simulink model "SoftFishHydrodynamicControl"  (R2020a)
settings: Solver=VariableStepAuto  StartTime=0.0  StopTime=40  FixedStep=1e-4  RelTol=1e-5
InitFcn:
  | initSoftFishHydrodynamicControl
values from neighbouring files (symbols this model uses):
  A33 = 0.25 * rho * pi * robotFinHeight * gamma    (= 8.1367249728)    [initSoftFishCocontraction.m]    (also in initSoftFishCocontractionControl.m; initSoftFishHydrodynamic.m; initSoftFishHydrodynamicControl.m)
  freq = 1    [initSoftFishCocontraction.m]    (also in initSoftFishCocontractionControl.m; initSoftFishHydrodynamic.m; initSoftFishHydrodynamicControl.m)
  modelElements = 5    [initSoftFishCocontraction.m]    (also in initSoftFishCocontractionControl.m; initSoftFishHydrodynamic.m; initSoftFishHydrodynamicControl.m)
  modelPressureCoefficient = pFinal(3)    [SoftFishSingleRun.m]    (also in SoftFishSingleRunWater.m)
  modelPressureLag = pFinal(5)    [SoftFishSingleRun.m]    (also in SoftFishSingleRunWater.m)
  modelPressureStiffness = pFinal(4)    [SoftFishSingleRun.m]    (also in SoftFishSingleRunWater.m)
  NoiseLevel = 0.05    [initSoftFishCocontractionControl.m]    (also in initSoftFishHydrodynamicControl.m)
  robotBlockLength = robotLength/modelElements    (= 0.028)    [initSoftFishCocontraction.m]    (also in initSoftFishCocontractionControl.m; initSoftFishHydrodynamic.m; initSoftFishHydrodynamicControl.m)
  robotBlockRevoluteRadius = 0.5 * robotBlockLength    (= 0.014)    [initSoftFishCocontraction.m]    (also in initSoftFishCocontractionControl.m; initSoftFishHydrodynamic.m; initSoftFishHydrodynamicControl.m)
  robotChamberHeight = 2e-2    (= 0.02)    [initSoftFishCocontraction.m]    (also in initSoftFishCocontractionControl.m; initSoftFishHydrodynamic.m; initSoftFishHydrodynamicControl.m)
  robotChamberWidth = 3e-2    (= 0.03)    [initSoftFishCocontraction.m]    (also in initSoftFishCocontractionControl.m; initSoftFishHydrodynamic.m; initSoftFishHydrodynamicControl.m)
  robotFinHeight = 7e-2    (= 0.07)    [initSoftFishCocontraction.m]    (also in initSoftFishCocontractionControl.m; initSoftFishHydrodynamic.m; initSoftFishHydrodynamicControl.m)
  robotFinWidth = 0.52*1e-3    (= 0.00052)    [initSoftFishCocontraction.m]    (also in initSoftFishCocontractionControl.m; initSoftFishHydrodynamic.m; initSoftFishHydrodynamicControl.m)
  robotLength = 112e-3*1.25    (= 0.14)    [initSoftFishCocontraction.m]    (also in initSoftFishCocontractionControl.m; initSoftFishHydrodynamic.m; initSoftFishHydrodynamicControl.m)
  robotMass = 2*42e-3    (= 0.084)    [initSoftFishCocontraction.m]    (also in initSoftFishCocontractionControl.m; initSoftFishHydrodynamic.m; initSoftFishHydrodynamicControl.m)
  Setpoint1 = 0.7    [initSoftFishCocontractionControl.m]    (also in initSoftFishHydrodynamicControl.m = 0.4)
  Setpoint2 = 1.4    [initSoftFishCocontractionControl.m]    (also in initSoftFishHydrodynamicControl.m = 0.6)
  Setpoint3 = 0.5    [initSoftFishCocontractionControl.m]    (also in initSoftFishHydrodynamicControl.m = 0.4)
  SwitchTime1 = 15    [initSoftFishCocontractionControl.m]    (also in initSoftFishHydrodynamicControl.m)
  SwitchTime2 = 25    [initSoftFishCocontractionControl.m]    (also in initSoftFishHydrodynamicControl.m = 30)
undefined symbols (not defined in the file or in its folder): X, Y, Z
libraries: nesl_utility x33, sm_lib x28, fl_lib x3, simulink x2
(part 2 of 2)

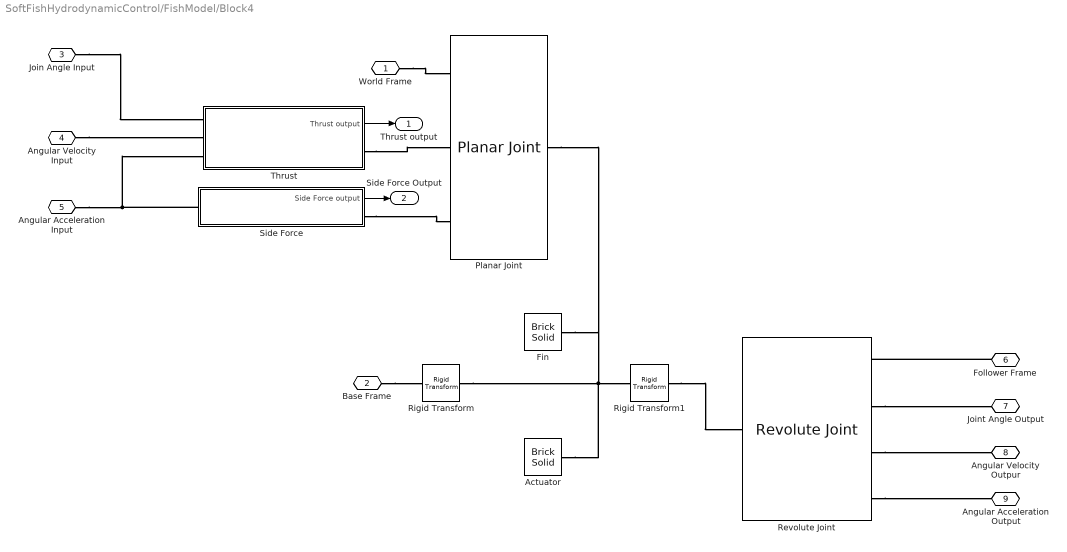
== system SoftFishHydrodynamicControl/FishModel/Block4 ==
  Actuator : sm_lib/Body Elements/Brick Solid  GraphicAmbientColor=[0.15 0.15 0.15 1.0]  BasedOnType=Mass  BrickDimensions=[robotLength/modelElements robotChamberWidth robotChamberHeight]  BrickDimensionUnits=m  CenterOfMass=[0 0 0]  CenterOfMassUnits=m  GraphicDiffuseColor=robotChamberColor  Density=1000  DensityUnits=kg/m^3  DoExposeReferenceFrame=on  GraphicEmissiveColor=[0.0 0.0 0.0 1.0]  ExportEntireGeometry=off  SerializedFrames=<Frames/>  MarkerShape=Sphere  MarkerSize=10  GraphicType=FromGeometry  InertiaType=CalculateFromGeometry  Mass=robotMass/modelElements  MassUnits=kg  MomentsOfInertia=[1 1 1]  MomentsOfInertiaUnits=kg*m^2  GraphicOpacity=1.0  ProductsOfInertia=[0 0 0]  ProductsOfInertiaUnits=kg*m^2  GraphicShininess=75  GraphicSpecularColor=[0.5 0.5 0.5 1.0]  GraphicVisPropType=SimpleVisualProperties
  Fin : sm_lib/Body Elements/Brick Solid  GraphicAmbientColor=[0.15 0.15 0.15 1.0]  BasedOnType=Density  BrickDimensions=[robotLength/modelElements robotFinWidth robotFinHeight]  BrickDimensionUnits=m  CenterOfMass=[0 0 0]  CenterOfMassUnits=m  GraphicDiffuseColor=[0.5 0.5 0.5]  Density=0  DensityUnits=kg/m^3  DoExposeReferenceFrame=on  GraphicEmissiveColor=[0.0 0.0 0.0 1.0]  ExportEntireGeometry=off  SerializedFrames=<Frames/>  MarkerShape=Sphere  MarkerSize=10  GraphicType=FromGeometry  InertiaType=CalculateFromGeometry  Mass=1  MassUnits=kg  MomentsOfInertia=[1 1 1]  MomentsOfInertiaUnits=kg*m^2  GraphicOpacity=1.0  ProductsOfInertia=[0 0 0]  ProductsOfInertiaUnits=kg*m^2  GraphicShininess=75  GraphicSpecularColor=[0.5 0.5 0.5 1.0]  GraphicVisPropType=SimpleVisualProperties
  Planar Joint : sm_lib/Joints/Planar Joint  JointMode=Normal  SenseConstraintForce=off  SenseConstraintForceX=off  SenseConstraintForceY=off  SenseConstraintForceZ=off  SenseConstraintTorque=off  SenseConstraintTorqueX=off  SenseConstraintTorqueY=off  SenseConstraintTorqueZ=off  SenseTotalForce=off  SenseTotalForceX=off  SenseTotalForceY=off  SenseTotalForceZ=off  SenseTotalTorque=off  SenseTotalTorqueX=off  SenseTotalTorqueY=off  SenseTotalTorqueZ=off  CompositeWrenchDir=FollowerOnBase  CompositeWrenchFrame=BaseFrame  PxEquilibriumPosition=0  PxEquilibriumPositionUnits=m  PxSpringStiffness=0  PxSpringStiffnessUnits=N/m  PxDampingCoefficient=0  PxDampingCoefficientUnits=N/(m/s)  PxTorqueActuationMode=InputTorque  PxMotionActuationMode=ComputedMotion  PxSensePosition=off  PxSenseVelocity=off  PxSenseAcceleration=off  PxSenseTorqueForce=off  PxSenseLowerLimitTorqueForce=off  PxSenseUpperLimitTorqueForce=off  PxLowerLimitSpecify=off  PxLowerLimitBound=-1  PxLowerLimitBoundUnits=m  PxLowerLimitStiffness=1e6  PxLowerLimitStiffnessUnits=N/m  PxLowerLimitDamping=1e3  PxLowerLimitDampingUnits=N/(m/s)  PxLowerLimitTransitionRegionWidth=1e-4  PxLowerLimitTransitionRegionWidthUnits=m  PxUpperLimitSpecify=off  PxUpperLimitBound=1  PxUpperLimitBoundUnits=m  PxUpperLimitStiffness=1e6  PxUpperLimitStiffnessUnits=N/m  PxUpperLimitDamping=1e3  PxUpperLimitDampingUnits=N/(m/s)  PxUpperLimitTransitionRegionWidth=1e-4  PxUpperLimitTransitionRegionWidthUnits=m  PxPositionTargetSpecify=off  PxPositionTargetPriority=High  PxPositionTargetValue=0  PxPositionTargetValueUnits=m  PxVelocityTargetSpecify=off  PxVelocityTargetPriority=High  PxVelocityTargetValue=0  PxVelocityTargetValueUnits=m/s  PyEquilibriumPosition=0  PyEquilibriumPositionUnits=m  PySpringStiffness=0  PySpringStiffnessUnits=N/m  PyDampingCoefficient=0  PyDampingCoefficientUnits=N/(m/s)  PyTorqueActuationMode=InputTorque  PyMotionActuationMode=ComputedMotion  PySensePosition=off  PySenseVelocity=off  PySenseAcceleration=off  PySenseTorqueForce=off  PySenseLowerLimitTorqueForce=off  PySenseUpperLimitTorqueForce=off  PyLowerLimitSpecify=off  PyLowerLimitBound=-1  PyLowerLimitBoundUnits=m  PyLowerLimitStiffness=1e6  PyLowerLimitStiffnessUnits=N/m  PyLowerLimitDamping=1e3  PyLowerLimitDampingUnits=N/(m/s)  PyLowerLimitTransitionRegionWidth=1e-4  PyLowerLimitTransitionRegionWidthUnits=m  PyUpperLimitSpecify=off  PyUpperLimitBound=1  PyUpperLimitBoundUnits=m  PyUpperLimitStiffness=1e6  PyUpperLimitStiffnessUnits=N/m  PyUpperLimitDamping=1e3  PyUpperLimitDampingUnits=N/(m/s)  PyUpperLimitTransitionRegionWidth=1e-4  PyUpperLimitTransitionRegionWidthUnits=m  PyPositionTargetSpecify=off  PyPositionTargetPriority=High  PyPositionTargetValue=0  PyPositionTargetValueUnits=m  PyVelocityTargetSpecify=off  PyVelocityTargetPriority=High  PyVelocityTargetValue=0  PyVelocityTargetValueUnits=m/s  RzEquilibriumPosition=0  RzEquilibriumPositionUnits=deg  RzSpringStiffness=0  RzSpringStiffnessUnits=N*m/deg  RzDampingCoefficient=0  RzDampingCoefficientUnits=N*m/(deg/s)  RzTorqueActuationMode=NoTorque  RzMotionActuationMode=ComputedMotion  RzSensePosition=off  RzSenseVelocity=off  RzSenseAcceleration=off  RzSenseTorqueForce=off  RzSenseLowerLimitTorqueForce=off  RzSenseUpperLimitTorqueForce=off  RzLowerLimitSpecify=off  RzLowerLimitBound=-90  RzLowerLimitBoundUnits=deg  RzLowerLimitStiffness=1e4  RzLowerLimitStiffnessUnits=N*m/deg  RzLowerLimitDamping=10  RzLowerLimitDampingUnits=N*m/(deg/s)  RzLowerLimitTransitionRegionWidth=0.1  RzLowerLimitTransitionRegionWidthUnits=deg  RzUpperLimitSpecify=off  RzUpperLimitBound=90  RzUpperLimitBoundUnits=deg  RzUpperLimitStiffness=1e4  RzUpperLimitStiffnessUnits=N*m/deg  RzUpperLimitDamping=10  RzUpperLimitDampingUnits=N*m/(deg/s)  RzUpperLimitTransitionRegionWidth=0.1  RzUpperLimitTransitionRegionWidthUnits=deg  RzPositionTargetSpecify=off  RzPositionTargetPriority=High  RzPositionTargetValue=0  RzPositionTargetValueUnits=deg  RzVelocityTargetSpecify=off  RzVelocityTargetPriority=High  RzVelocityTargetValue=0  RzVelocityTargetValueUnits=deg/s
  Revolute Joint : sm_lib/Joints/Revolute Joint  JointMode=Normal  SenseConstraintForce=off  SenseConstraintForceX=off  SenseConstraintForceY=off  SenseConstraintForceZ=off  SenseConstraintTorque=off  SenseConstraintTorqueX=off  SenseConstraintTorqueY=off  SenseConstraintTorqueZ=off  SenseTotalForce=off  SenseTotalForceX=off  SenseTotalForceY=off  SenseTotalForceZ=off  SenseTotalTorque=off  SenseTotalTorqueX=off  SenseTotalTorqueY=off  SenseTotalTorqueZ=off  CompositeWrenchDir=FollowerOnBase  CompositeWrenchFrame=BaseFrame  EquilibriumPosition=0  EquilibriumPositionUnits=deg  SpringStiffness=robotFinStiffness  SpringStiffnessUnits=N*m/rad  DampingCoefficient=0  DampingCoefficientUnits=N*m/(deg/s)  TorqueActuationMode=NoTorque  MotionActuationMode=ComputedMotion  SensePosition=on  SenseVelocity=on  SenseAcceleration=on  SenseTorqueForce=off  SenseLowerLimitTorqueForce=off  SenseUpperLimitTorqueForce=off  LowerLimitSpecify=off  LowerLimitBound=-90  LowerLimitBoundUnits=deg  LowerLimitStiffness=1e4  LowerLimitStiffnessUnits=N*m/deg  LowerLimitDamping=10  LowerLimitDampingUnits=N*m/(deg/s)  LowerLimitTransitionRegionWidth=0.1  LowerLimitTransitionRegionWidthUnits=deg  UpperLimitSpecify=off  UpperLimitBound=90  UpperLimitBoundUnits=deg  UpperLimitStiffness=1e4  UpperLimitStiffnessUnits=N*m/deg  UpperLimitDamping=10  UpperLimitDampingUnits=N*m/(deg/s)  UpperLimitTransitionRegionWidth=0.1  UpperLimitTransitionRegionWidthUnits=deg  PositionTargetSpecify=off  PositionTargetPriority=High  PositionTargetValue=0  PositionTargetValueUnits=deg  VelocityTargetSpecify=off  VelocityTargetPriority=High  VelocityTargetValue=0  VelocityTargetValueUnits=deg/s
  Rigid Transform : sm_lib/Frames and Transforms/Rigid Transform  TranslationMethod=StandardAxis  TranslationStandardOffset=robotLength*0.5/modelElements  TranslationLengthUnit=m  TranslationStandardAxis=+X  TranslationCartesianOffset=[0 0 0]  TranslationROffset=0  TranslationROffsetUnits=m  TranslationZOffset=0  TranslationZOffsetUnits=m  TranslationThetaOffset=0  TranslationThetaOffsetUnits=deg  RotationMethod=None  RotationAngleUnits=deg  RotationStandardAxis=+Z  RotationAngle=0.0  RotationArbitraryAxis=[0 0 1]  FollAlignAxisA=+X  BaseAlignAxisA=+Y  FollAlignAxisB=+Y  BaseAlignAxisB=+Z  RotationSequenceAxes=FollowerAxes  RotationSequence=XYX  RotationSequenceAngles=[0 0 0]  RotationSequenceAnglesUnits=deg  RotationMatrix=[1 0 0; 0 1 0; 0 0 1]
  Rigid Transform1 : sm_lib/Frames and Transforms/Rigid Transform  TranslationMethod=StandardAxis  TranslationStandardOffset=robotLength*0.5/modelElements  TranslationLengthUnit=m  TranslationStandardAxis=+X  TranslationCartesianOffset=[0 0 0]  TranslationROffset=0  TranslationROffsetUnits=m  TranslationZOffset=0  TranslationZOffsetUnits=m  TranslationThetaOffset=0  TranslationThetaOffsetUnits=deg  RotationMethod=None  RotationAngleUnits=deg  RotationStandardAxis=+Z  RotationAngle=0.0  RotationArbitraryAxis=[0 0 1]  FollAlignAxisA=+X  BaseAlignAxisA=+Y  FollAlignAxisB=+Y  BaseAlignAxisB=+Z  RotationSequenceAxes=FollowerAxes  RotationSequence=XYX  RotationSequenceAngles=[0 0 0]  RotationSequenceAnglesUnits=deg  RotationMatrix=[1 0 0; 0 1 0; 0 0 1]
  Side Force : Subsystem
  Thrust : Subsystem
  World Frame : PMIOPort  Side=Left
  Base Frame : PMIOPort  Port=2  Side=Left
  Join Angle Input : PMIOPort  Port=3  Side=Left
  Angular Velocity Input : PMIOPort  Port=4  Side=Left
  Angular Acceleration Input : PMIOPort  Port=5  Side=Left
  Follower Frame : PMIOPort  Port=6  Side=Right
  "Joint Angle Output " : PMIOPort  Port=7  Side=Right
  Angular Velocity Outpur : PMIOPort  Port=8  Side=Right
  Angular Acceleration Output : PMIOPort  Port=9  Side=Right
  Thrust output : Outport
  Side Force Output : Outport  Port=2
  wires:
  Thrust/1(Thrust output) -> Thrust output/1
  Side Force/1(Side Force output) -> Side Force Output/1
  connections:
  Base Frame/RConn1 -- Rigid Transform/LConn1
  Rigid Transform/RConn1 -- Actuator/RConn1 -- Rigid Transform1/LConn1 -- Planar Joint/RConn1 -- Fin/RConn1
  Rigid Transform1/RConn1 -- Revolute Joint/LConn1
  Follower Frame/RConn1 -- Revolute Joint/RConn1
  Revolute Joint/RConn2 -- "Joint Angle Output "/RConn1
  Revolute Joint/RConn3 -- Angular Velocity Outpur/RConn1
  Revolute Joint/RConn4 -- Angular Acceleration Output/RConn1
  World Frame/RConn1 -- Planar Joint/LConn1
  Angular Acceleration Input/RConn1 -- Thrust/LConn3 -- Side Force/LConn1
  Side Force/RConn1 -- Planar Joint/LConn3
  Thrust/RConn1 -- Planar Joint/LConn2
  Join Angle Input/RConn1 -- Thrust/LConn1
  Angular Velocity Input/RConn1 -- Thrust/LConn2

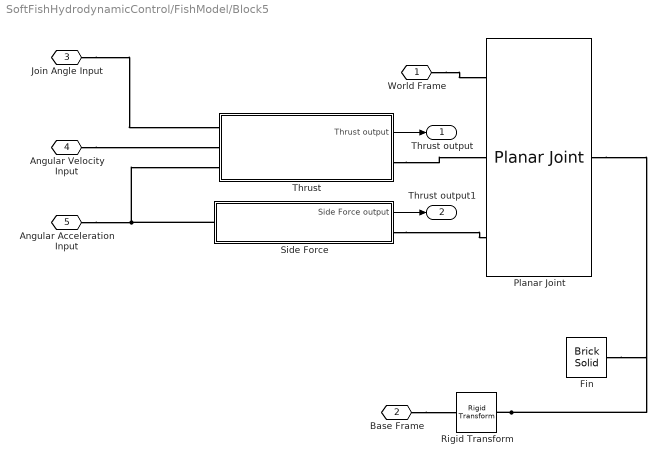
== system SoftFishHydrodynamicControl/FishModel/Block5 ==
  Fin : sm_lib/Body Elements/Brick Solid  GraphicAmbientColor=[0.15 0.15 0.15 1.0]  BasedOnType=Density  BrickDimensions=[2*robotBlockLength robotFinWidth robotFinHeight]  BrickDimensionUnits=m  CenterOfMass=[0 0 0]  CenterOfMassUnits=m  GraphicDiffuseColor=[0.5 0.5 0.5]  Density=0.92  DensityUnits=g/cm^3  DoExposeReferenceFrame=on  GraphicEmissiveColor=[0.0 0.0 0.0 1.0]  ExportEntireGeometry=off  SerializedFrames=<Frames/>  MarkerShape=Sphere  MarkerSize=10  GraphicType=FromGeometry  InertiaType=CalculateFromGeometry  Mass=1  MassUnits=kg  MomentsOfInertia=[1 1 1]  MomentsOfInertiaUnits=kg*m^2  GraphicOpacity=1.0  ProductsOfInertia=[0 0 0]  ProductsOfInertiaUnits=kg*m^2  GraphicShininess=75  GraphicSpecularColor=[0.5 0.5 0.5 1.0]  GraphicVisPropType=SimpleVisualProperties
  Planar Joint : sm_lib/Joints/Planar Joint  JointMode=Normal  SenseConstraintForce=off  SenseConstraintForceX=off  SenseConstraintForceY=off  SenseConstraintForceZ=off  SenseConstraintTorque=off  SenseConstraintTorqueX=off  SenseConstraintTorqueY=off  SenseConstraintTorqueZ=off  SenseTotalForce=off  SenseTotalForceX=off  SenseTotalForceY=off  SenseTotalForceZ=off  SenseTotalTorque=off  SenseTotalTorqueX=off  SenseTotalTorqueY=off  SenseTotalTorqueZ=off  CompositeWrenchDir=FollowerOnBase  CompositeWrenchFrame=BaseFrame  PxEquilibriumPosition=0  PxEquilibriumPositionUnits=m  PxSpringStiffness=0  PxSpringStiffnessUnits=N/m  PxDampingCoefficient=0  PxDampingCoefficientUnits=N/(m/s)  PxTorqueActuationMode=InputTorque  PxMotionActuationMode=ComputedMotion  PxSensePosition=off  PxSenseVelocity=off  PxSenseAcceleration=off  PxSenseTorqueForce=off  PxSenseLowerLimitTorqueForce=off  PxSenseUpperLimitTorqueForce=off  PxLowerLimitSpecify=off  PxLowerLimitBound=-1  PxLowerLimitBoundUnits=m  PxLowerLimitStiffness=1e6  PxLowerLimitStiffnessUnits=N/m  PxLowerLimitDamping=1e3  PxLowerLimitDampingUnits=N/(m/s)  PxLowerLimitTransitionRegionWidth=1e-4  PxLowerLimitTransitionRegionWidthUnits=m  PxUpperLimitSpecify=off  PxUpperLimitBound=1  PxUpperLimitBoundUnits=m  PxUpperLimitStiffness=1e6  PxUpperLimitStiffnessUnits=N/m  PxUpperLimitDamping=1e3  PxUpperLimitDampingUnits=N/(m/s)  PxUpperLimitTransitionRegionWidth=1e-4  PxUpperLimitTransitionRegionWidthUnits=m  PxPositionTargetSpecify=off  PxPositionTargetPriority=High  PxPositionTargetValue=0  PxPositionTargetValueUnits=m  PxVelocityTargetSpecify=off  PxVelocityTargetPriority=High  PxVelocityTargetValue=0  PxVelocityTargetValueUnits=m/s  PyEquilibriumPosition=0  PyEquilibriumPositionUnits=m  PySpringStiffness=0  PySpringStiffnessUnits=N/m  PyDampingCoefficient=0  PyDampingCoefficientUnits=N/(m/s)  PyTorqueActuationMode=InputTorque  PyMotionActuationMode=ComputedMotion  PySensePosition=off  PySenseVelocity=off  PySenseAcceleration=off  PySenseTorqueForce=off  PySenseLowerLimitTorqueForce=off  PySenseUpperLimitTorqueForce=off  PyLowerLimitSpecify=off  PyLowerLimitBound=-1  PyLowerLimitBoundUnits=m  PyLowerLimitStiffness=1e6  PyLowerLimitStiffnessUnits=N/m  PyLowerLimitDamping=1e3  PyLowerLimitDampingUnits=N/(m/s)  PyLowerLimitTransitionRegionWidth=1e-4  PyLowerLimitTransitionRegionWidthUnits=m  PyUpperLimitSpecify=off  PyUpperLimitBound=1  PyUpperLimitBoundUnits=m  PyUpperLimitStiffness=1e6  PyUpperLimitStiffnessUnits=N/m  PyUpperLimitDamping=1e3  PyUpperLimitDampingUnits=N/(m/s)  PyUpperLimitTransitionRegionWidth=1e-4  PyUpperLimitTransitionRegionWidthUnits=m  PyPositionTargetSpecify=off  PyPositionTargetPriority=High  PyPositionTargetValue=0  PyPositionTargetValueUnits=m  PyVelocityTargetSpecify=off  PyVelocityTargetPriority=High  PyVelocityTargetValue=0  PyVelocityTargetValueUnits=m/s  RzEquilibriumPosition=0  RzEquilibriumPositionUnits=deg  RzSpringStiffness=0  RzSpringStiffnessUnits=N*m/deg  RzDampingCoefficient=0  RzDampingCoefficientUnits=N*m/(deg/s)  RzTorqueActuationMode=NoTorque  RzMotionActuationMode=ComputedMotion  RzSensePosition=off  RzSenseVelocity=off  RzSenseAcceleration=off  RzSenseTorqueForce=off  RzSenseLowerLimitTorqueForce=off  RzSenseUpperLimitTorqueForce=off  RzLowerLimitSpecify=off  RzLowerLimitBound=-90  RzLowerLimitBoundUnits=deg  RzLowerLimitStiffness=1e4  RzLowerLimitStiffnessUnits=N*m/deg  RzLowerLimitDamping=10  RzLowerLimitDampingUnits=N*m/(deg/s)  RzLowerLimitTransitionRegionWidth=0.1  RzLowerLimitTransitionRegionWidthUnits=deg  RzUpperLimitSpecify=off  RzUpperLimitBound=90  RzUpperLimitBoundUnits=deg  RzUpperLimitStiffness=1e4  RzUpperLimitStiffnessUnits=N*m/deg  RzUpperLimitDamping=10  RzUpperLimitDampingUnits=N*m/(deg/s)  RzUpperLimitTransitionRegionWidth=0.1  RzUpperLimitTransitionRegionWidthUnits=deg  RzPositionTargetSpecify=off  RzPositionTargetPriority=High  RzPositionTargetValue=0  RzPositionTargetValueUnits=deg  RzVelocityTargetSpecify=off  RzVelocityTargetPriority=High  RzVelocityTargetValue=0  RzVelocityTargetValueUnits=deg/s
  Rigid Transform : sm_lib/Frames and Transforms/Rigid Transform  TranslationMethod=StandardAxis  TranslationStandardOffset=robotLength*0.5/modelElements  TranslationLengthUnit=m  TranslationStandardAxis=+X  TranslationCartesianOffset=[0 0 0]  TranslationROffset=0  TranslationROffsetUnits=m  TranslationZOffset=0  TranslationZOffsetUnits=m  TranslationThetaOffset=0  TranslationThetaOffsetUnits=deg  RotationMethod=None  RotationAngleUnits=deg  RotationStandardAxis=+Z  RotationAngle=0.0  RotationArbitraryAxis=[0 0 1]  FollAlignAxisA=+X  BaseAlignAxisA=+Y  FollAlignAxisB=+Y  BaseAlignAxisB=+Z  RotationSequenceAxes=FollowerAxes  RotationSequence=XYX  RotationSequenceAngles=[0 0 0]  RotationSequenceAnglesUnits=deg  RotationMatrix=[1 0 0; 0 1 0; 0 0 1]
  Side Force : Subsystem
  Thrust : Subsystem
  World Frame : PMIOPort  Side=Left
  Base Frame : PMIOPort  Port=2  Side=Left
  Join Angle Input : PMIOPort  Port=3  Side=Left
  Angular Velocity Input : PMIOPort  Port=4  Side=Left
  Angular Acceleration Input : PMIOPort  Port=5  Side=Left
  Thrust output : Outport
  Thrust output1 : Outport  Port=2
  wires:
  Thrust/1(Thrust output) -> Thrust output/1
  Side Force/1(Side Force output) -> Thrust output1/1
  connections:
  Base Frame/RConn1 -- Rigid Transform/LConn1
  Rigid Transform/RConn1 -- Planar Joint/RConn1 -- Fin/RConn1
  World Frame/RConn1 -- Planar Joint/LConn1
  Angular Acceleration Input/RConn1 -- Thrust/LConn3 -- Side Force/LConn1
  Side Force/RConn1 -- Planar Joint/LConn3
  Thrust/RConn1 -- Planar Joint/LConn2
  Join Angle Input/RConn1 -- Thrust/LConn1
  Angular Velocity Input/RConn1 -- Thrust/LConn2

== system SoftFishHydrodynamicControl/Peak Extractor/Triggered Subsystem ==
  In1 : Inport
  Trigger : TriggerPort  TriggerType=either  VariantControl=Variant
  Out1 : Outport
  wires:
  In1/1 -> Out1/1

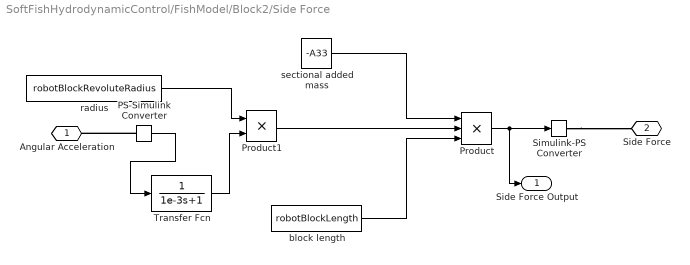
== system SoftFishHydrodynamicControl/FishModel/Block2/Side Force ==
  PS-Simulink Converter : nesl_utility/PS-Simulink Converter  PhysicalDomain=network_engine_domain  SubClassName=ps_output  LeftPortType=input  RightPortType=output  PseudoPeriodic=off  Frequencies=[]  Unit=inherit  AffineConversion=off
  Product : Product  Inputs=3
  Product1 : Product
  Simulink-PS Converter : nesl_utility/Simulink-PS Converter  PhysicalDomain=network_engine_domain  SubClassName=ps_input  LeftPortType=input  RightPortType=output  PseudoPeriodic=off  Frequencies=[]  NoiseDistribution=none  NoiseParameters=[]  Unit=1  AffineConversion=off  FilteringAndDerivatives=provide  SimscapeFilterOrder=1  InputFilterTimeConstant=0.001  UdotUserProvided=0
  Transfer Fcn : TransferFcn  Denominator=[1e-3 1]
  block length : Constant  Value=robotBlockLength
  radius : Constant  Value=robotBlockRevoluteRadius
  sectional added mass : Constant  Value=-A33
  Angular Acceleration : PMIOPort  Side=Left
  Side Force : PMIOPort  Port=2  Side=Right
  Side Force Output : Outport
  wires:
  sectional added mass/1 -> Product/1
  block length/1 -> Product/3
  Product/1 -> Side Force Output/1, Simulink-PS Converter/1
  Product1/1 -> Product/2
  radius/1 -> Product1/1
  PS-Simulink Converter/1 -> Transfer Fcn/1
  Transfer Fcn/1 -> Product1/2
  connections:
  Simulink-PS Converter/RConn1 -- Side Force/RConn1
  PS-Simulink Converter/LConn1 -- Angular Acceleration/RConn1

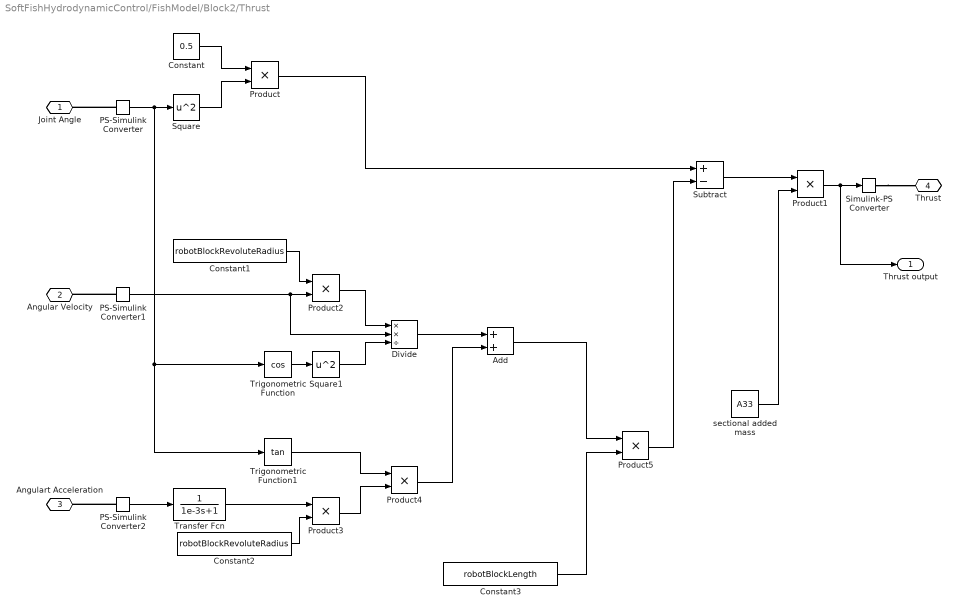
== system SoftFishHydrodynamicControl/FishModel/Block2/Thrust ==
  Add : Sum
  Constant : Constant  Value=0.5
  Constant1 : Constant  Value=robotBlockRevoluteRadius
  Constant2 : Constant  Value=robotBlockRevoluteRadius
  Constant3 : Constant  Value=robotBlockLength
  Divide : Product  Inputs=**/
  PS-Simulink Converter : nesl_utility/PS-Simulink Converter  PhysicalDomain=network_engine_domain  SubClassName=ps_output  LeftPortType=input  RightPortType=output  PseudoPeriodic=off  Frequencies=[]  Unit=inherit  AffineConversion=off
  PS-Simulink Converter1 : nesl_utility/PS-Simulink Converter  PhysicalDomain=network_engine_domain  SubClassName=ps_output  LeftPortType=input  RightPortType=output  PseudoPeriodic=off  Frequencies=[]  Unit=inherit  AffineConversion=off
  PS-Simulink Converter2 : nesl_utility/PS-Simulink Converter  PhysicalDomain=network_engine_domain  SubClassName=ps_output  LeftPortType=input  RightPortType=output  PseudoPeriodic=off  Frequencies=[]  Unit=inherit  AffineConversion=off
  Product{,1..5} (6 alike) : Product
  Simulink-PS Converter : nesl_utility/Simulink-PS Converter  PhysicalDomain=network_engine_domain  SubClassName=ps_input  LeftPortType=input  RightPortType=output  PseudoPeriodic=off  Frequencies=[]  NoiseDistribution=none  NoiseParameters=[]  Unit=1  AffineConversion=off  FilteringAndDerivatives=provide  SimscapeFilterOrder=1  InputFilterTimeConstant=0.001  UdotUserProvided=0
  Square : Math  Operator=square  SaturateOnIntegerOverflow=on
  Square1 : Math  Operator=square  SaturateOnIntegerOverflow=on
  Subtract : Sum  Inputs=+-
  Transfer Fcn : TransferFcn  Denominator=[1e-3 1]
  Trigonometric Function : Trigonometry  Operator=cos
  Trigonometric Function1 : Trigonometry  Operator=tan
  sectional added mass : Constant  Value=A33
  Joint Angle : PMIOPort  Side=Left
  Angular Velocity : PMIOPort  Port=2  Side=Left
  Angulart Acceleration : PMIOPort  Port=3  Side=Left
  Thrust : PMIOPort  Port=4  Side=Right
  Thrust output : Outport
  wires:
  Constant/1 -> Product/1
  Square/1 -> Product/2
  sectional added mass/1 -> Product1/2
  Subtract/1 -> Product1/1
  Product/1 -> Subtract/1
  Trigonometric Function/1 -> Square1/1
  PS-Simulink Converter1/1 -> Divide/2, Product2/2
  Product2/1 -> Divide/1
  Square1/1 -> Divide/3
  Divide/1 -> Add/1
  Constant1/1 -> Product2/1
  PS-Simulink Converter2/1 -> Transfer Fcn/1
  Constant2/1 -> Product3/2
  Product3/1 -> Product4/2
  Trigonometric Function1/1 -> Product4/1
  Product4/1 -> Add/2
  Add/1 -> Product5/1
  Constant3/1 -> Product5/2
  Product5/1 -> Subtract/2
  Product1/1 -> Thrust output/1, Simulink-PS Converter/1
  Transfer Fcn/1 -> Product3/1
  PS-Simulink Converter/1 -> Trigonometric Function1/1, Trigonometric Function/1, Square/1
  connections:
  PS-Simulink Converter/LConn1 -- Joint Angle/RConn1
  PS-Simulink Converter2/LConn1 -- Angulart Acceleration/RConn1
  PS-Simulink Converter1/LConn1 -- Angular Velocity/RConn1
  Simulink-PS Converter/RConn1 -- Thrust/RConn1

== system SoftFishHydrodynamicControl/FishModel/Block3/Side Force ==
  PS-Simulink Converter : nesl_utility/PS-Simulink Converter  PhysicalDomain=network_engine_domain  SubClassName=ps_output  LeftPortType=input  RightPortType=output  PseudoPeriodic=off  Frequencies=[]  Unit=inherit  AffineConversion=off
  Product : Product  Inputs=3
  Product1 : Product
  Simulink-PS Converter : nesl_utility/Simulink-PS Converter  PhysicalDomain=network_engine_domain  SubClassName=ps_input  LeftPortType=input  RightPortType=output  PseudoPeriodic=off  Frequencies=[]  NoiseDistribution=none  NoiseParameters=[]  Unit=1  AffineConversion=off  FilteringAndDerivatives=provide  SimscapeFilterOrder=1  InputFilterTimeConstant=0.001  UdotUserProvided=0
  Transfer Fcn : TransferFcn  Denominator=[1e-3 1]
  block length : Constant  Value=robotBlockLength
  radius : Constant  Value=robotBlockRevoluteRadius
  sectional added mass : Constant  Value=-A33
  Angular Acceleration : PMIOPort  Side=Left
  Side Force : PMIOPort  Port=2  Side=Right
  Side Force output : Outport
  wires:
  sectional added mass/1 -> Product/1
  block length/1 -> Product/3
  Product/1 -> Side Force output/1, Simulink-PS Converter/1
  Product1/1 -> Product/2
  radius/1 -> Product1/1
  PS-Simulink Converter/1 -> Transfer Fcn/1
  Transfer Fcn/1 -> Product1/2
  connections:
  Simulink-PS Converter/RConn1 -- Side Force/RConn1
  PS-Simulink Converter/LConn1 -- Angular Acceleration/RConn1

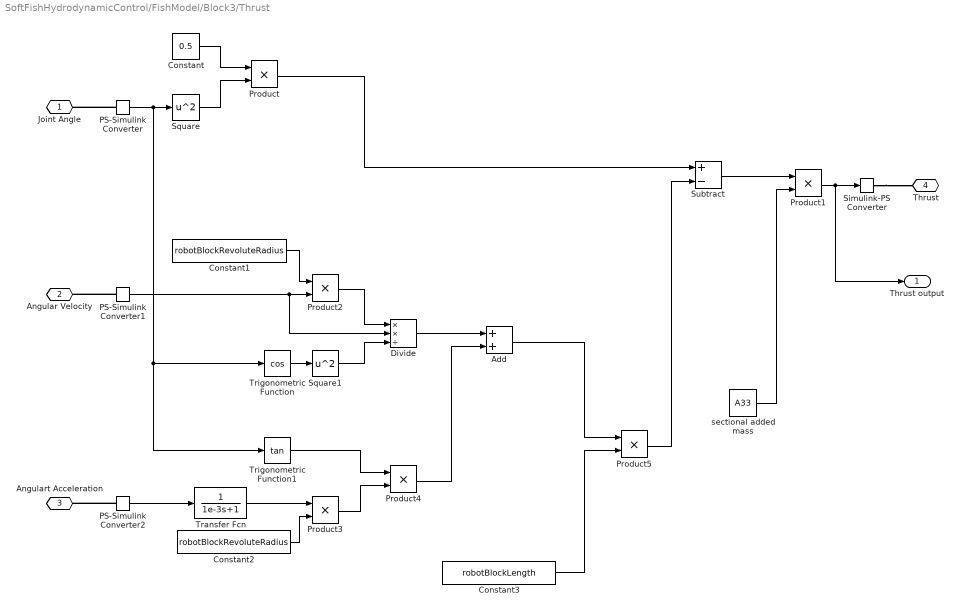
== system SoftFishHydrodynamicControl/FishModel/Block3/Thrust ==
  Add : Sum
  Constant : Constant  Value=0.5
  Constant1 : Constant  Value=robotBlockRevoluteRadius
  Constant2 : Constant  Value=robotBlockRevoluteRadius
  Constant3 : Constant  Value=robotBlockLength
  Divide : Product  Inputs=**/
  PS-Simulink Converter : nesl_utility/PS-Simulink Converter  PhysicalDomain=network_engine_domain  SubClassName=ps_output  LeftPortType=input  RightPortType=output  PseudoPeriodic=off  Frequencies=[]  Unit=inherit  AffineConversion=off
  PS-Simulink Converter1 : nesl_utility/PS-Simulink Converter  PhysicalDomain=network_engine_domain  SubClassName=ps_output  LeftPortType=input  RightPortType=output  PseudoPeriodic=off  Frequencies=[]  Unit=inherit  AffineConversion=off
  PS-Simulink Converter2 : nesl_utility/PS-Simulink Converter  PhysicalDomain=network_engine_domain  SubClassName=ps_output  LeftPortType=input  RightPortType=output  PseudoPeriodic=off  Frequencies=[]  Unit=inherit  AffineConversion=off
  Product{,1..5} (6 alike) : Product
  Simulink-PS Converter : nesl_utility/Simulink-PS Converter  PhysicalDomain=network_engine_domain  SubClassName=ps_input  LeftPortType=input  RightPortType=output  PseudoPeriodic=off  Frequencies=[]  NoiseDistribution=none  NoiseParameters=[]  Unit=1  AffineConversion=off  FilteringAndDerivatives=provide  SimscapeFilterOrder=1  InputFilterTimeConstant=0.001  UdotUserProvided=0
  Square : Math  Operator=square  SaturateOnIntegerOverflow=on
  Square1 : Math  Operator=square  SaturateOnIntegerOverflow=on
  Subtract : Sum  Inputs=+-
  Transfer Fcn : TransferFcn  Denominator=[1e-3 1]
  Trigonometric Function : Trigonometry  Operator=cos
  Trigonometric Function1 : Trigonometry  Operator=tan
  sectional added mass : Constant  Value=A33
  Joint Angle : PMIOPort  Side=Left
  Angular Velocity : PMIOPort  Port=2  Side=Left
  Angulart Acceleration : PMIOPort  Port=3  Side=Left
  Thrust : PMIOPort  Port=4  Side=Right
  Thrust output : Outport
  wires:
  Constant/1 -> Product/1
  Square/1 -> Product/2
  sectional added mass/1 -> Product1/2
  Subtract/1 -> Product1/1
  Product/1 -> Subtract/1
  Trigonometric Function/1 -> Square1/1
  PS-Simulink Converter1/1 -> Divide/2, Product2/2
  Product2/1 -> Divide/1
  Square1/1 -> Divide/3
  Divide/1 -> Add/1
  Constant1/1 -> Product2/1
  PS-Simulink Converter2/1 -> Transfer Fcn/1
  Constant2/1 -> Product3/2
  Product3/1 -> Product4/2
  Trigonometric Function1/1 -> Product4/1
  Product4/1 -> Add/2
  Add/1 -> Product5/1
  Constant3/1 -> Product5/2
  Product5/1 -> Subtract/2
  Product1/1 -> Thrust output/1, Simulink-PS Converter/1
  Transfer Fcn/1 -> Product3/1
  PS-Simulink Converter/1 -> Trigonometric Function1/1, Trigonometric Function/1, Square/1
  connections:
  PS-Simulink Converter/LConn1 -- Joint Angle/RConn1
  PS-Simulink Converter2/LConn1 -- Angulart Acceleration/RConn1
  PS-Simulink Converter1/LConn1 -- Angular Velocity/RConn1
  Simulink-PS Converter/RConn1 -- Thrust/RConn1

== system SoftFishHydrodynamicControl/FishModel/Block4/Side Force ==
  PS-Simulink Converter : nesl_utility/PS-Simulink Converter  PhysicalDomain=network_engine_domain  SubClassName=ps_output  LeftPortType=input  RightPortType=output  PseudoPeriodic=off  Frequencies=[]  Unit=inherit  AffineConversion=off
  Product : Product  Inputs=3
  Product1 : Product
  Simulink-PS Converter : nesl_utility/Simulink-PS Converter  PhysicalDomain=network_engine_domain  SubClassName=ps_input  LeftPortType=input  RightPortType=output  PseudoPeriodic=off  Frequencies=[]  NoiseDistribution=none  NoiseParameters=[]  Unit=1  AffineConversion=off  FilteringAndDerivatives=provide  SimscapeFilterOrder=1  InputFilterTimeConstant=0.001  UdotUserProvided=0
  Transfer Fcn : TransferFcn  Denominator=[1e-3 1]
  block length : Constant  Value=robotBlockLength
  radius : Constant  Value=robotBlockRevoluteRadius
  sectional added mass : Constant  Value=-A33
  Angular Acceleration : PMIOPort  Side=Left
  Side Force : PMIOPort  Port=2  Side=Right
  Side Force output : Outport
  wires:
  sectional added mass/1 -> Product/1
  block length/1 -> Product/3
  Product/1 -> Side Force output/1, Simulink-PS Converter/1
  Product1/1 -> Product/2
  radius/1 -> Product1/1
  PS-Simulink Converter/1 -> Transfer Fcn/1
  Transfer Fcn/1 -> Product1/2
  connections:
  Simulink-PS Converter/RConn1 -- Side Force/RConn1
  PS-Simulink Converter/LConn1 -- Angular Acceleration/RConn1

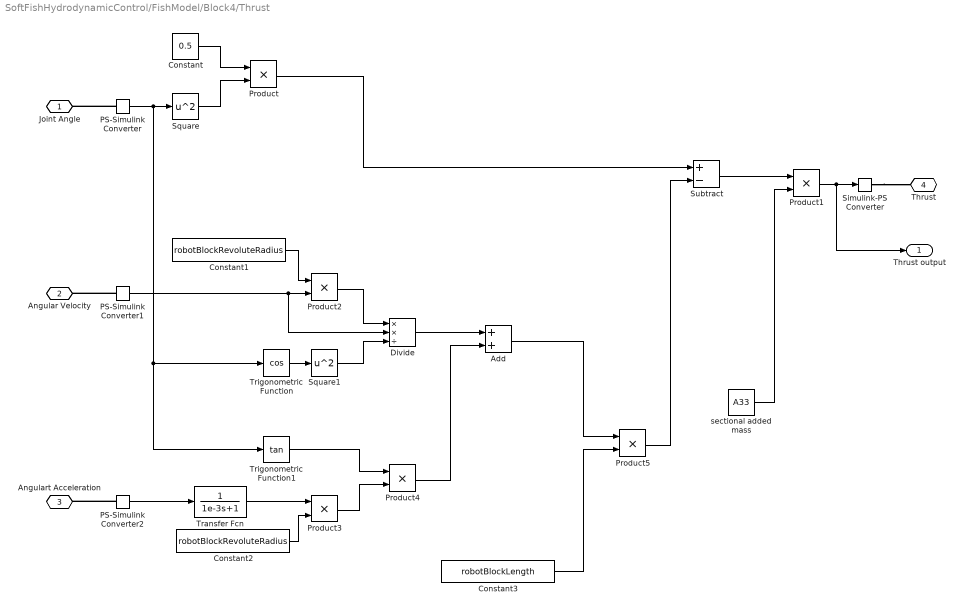
== system SoftFishHydrodynamicControl/FishModel/Block4/Thrust ==
  Add : Sum
  Constant : Constant  Value=0.5
  Constant1 : Constant  Value=robotBlockRevoluteRadius
  Constant2 : Constant  Value=robotBlockRevoluteRadius
  Constant3 : Constant  Value=robotBlockLength
  Divide : Product  Inputs=**/
  PS-Simulink Converter : nesl_utility/PS-Simulink Converter  PhysicalDomain=network_engine_domain  SubClassName=ps_output  LeftPortType=input  RightPortType=output  PseudoPeriodic=off  Frequencies=[]  Unit=inherit  AffineConversion=off
  PS-Simulink Converter1 : nesl_utility/PS-Simulink Converter  PhysicalDomain=network_engine_domain  SubClassName=ps_output  LeftPortType=input  RightPortType=output  PseudoPeriodic=off  Frequencies=[]  Unit=inherit  AffineConversion=off
  PS-Simulink Converter2 : nesl_utility/PS-Simulink Converter  PhysicalDomain=network_engine_domain  SubClassName=ps_output  LeftPortType=input  RightPortType=output  PseudoPeriodic=off  Frequencies=[]  Unit=inherit  AffineConversion=off
  Product{,1..5} (6 alike) : Product
  Simulink-PS Converter : nesl_utility/Simulink-PS Converter  PhysicalDomain=network_engine_domain  SubClassName=ps_input  LeftPortType=input  RightPortType=output  PseudoPeriodic=off  Frequencies=[]  NoiseDistribution=none  NoiseParameters=[]  Unit=1  AffineConversion=off  FilteringAndDerivatives=provide  SimscapeFilterOrder=1  InputFilterTimeConstant=0.001  UdotUserProvided=0
  Square : Math  Operator=square  SaturateOnIntegerOverflow=on
  Square1 : Math  Operator=square  SaturateOnIntegerOverflow=on
  Subtract : Sum  Inputs=+-
  Transfer Fcn : TransferFcn  Denominator=[1e-3 1]
  Trigonometric Function : Trigonometry  Operator=cos
  Trigonometric Function1 : Trigonometry  Operator=tan
  sectional added mass : Constant  Value=A33
  Joint Angle : PMIOPort  Side=Left
  Angular Velocity : PMIOPort  Port=2  Side=Left
  Angulart Acceleration : PMIOPort  Port=3  Side=Left
  Thrust : PMIOPort  Port=4  Side=Right
  Thrust output : Outport
  wires:
  Constant/1 -> Product/1
  Square/1 -> Product/2
  sectional added mass/1 -> Product1/2
  Subtract/1 -> Product1/1
  Product/1 -> Subtract/1
  Trigonometric Function/1 -> Square1/1
  PS-Simulink Converter1/1 -> Divide/2, Product2/2
  Product2/1 -> Divide/1
  Square1/1 -> Divide/3
  Divide/1 -> Add/1
  Constant1/1 -> Product2/1
  PS-Simulink Converter2/1 -> Transfer Fcn/1
  Constant2/1 -> Product3/2
  Product3/1 -> Product4/2
  Trigonometric Function1/1 -> Product4/1
  Product4/1 -> Add/2
  Add/1 -> Product5/1
  Constant3/1 -> Product5/2
  Product5/1 -> Subtract/2
  Product1/1 -> Thrust output/1, Simulink-PS Converter/1
  Transfer Fcn/1 -> Product3/1
  PS-Simulink Converter/1 -> Trigonometric Function1/1, Trigonometric Function/1, Square/1
  connections:
  PS-Simulink Converter/LConn1 -- Joint Angle/RConn1
  PS-Simulink Converter2/LConn1 -- Angulart Acceleration/RConn1
  PS-Simulink Converter1/LConn1 -- Angular Velocity/RConn1
  Simulink-PS Converter/RConn1 -- Thrust/RConn1

== system SoftFishHydrodynamicControl/FishModel/Block5/Side Force ==
  PS-Simulink Converter : nesl_utility/PS-Simulink Converter  PhysicalDomain=network_engine_domain  SubClassName=ps_output  LeftPortType=input  RightPortType=output  PseudoPeriodic=off  Frequencies=[]  Unit=inherit  AffineConversion=off
  Product : Product  Inputs=3
  Product1 : Product
  Simulink-PS Converter : nesl_utility/Simulink-PS Converter  PhysicalDomain=network_engine_domain  SubClassName=ps_input  LeftPortType=input  RightPortType=output  PseudoPeriodic=off  Frequencies=[]  NoiseDistribution=none  NoiseParameters=[]  Unit=1  AffineConversion=off  FilteringAndDerivatives=provide  SimscapeFilterOrder=1  InputFilterTimeConstant=0.001  UdotUserProvided=0
  Transfer Fcn : TransferFcn  Denominator=[1e-3 1]
  block length : Constant  Value=robotBlockLength
  radius : Constant  Value=robotBlockRevoluteRadius
  sectional added mass : Constant  Value=-A33
  Angular Acceleration : PMIOPort  Side=Left
  Side Force : PMIOPort  Port=2  Side=Right
  Side Force output : Outport
  wires:
  sectional added mass/1 -> Product/1
  block length/1 -> Product/3
  Product/1 -> Side Force output/1, Simulink-PS Converter/1
  Product1/1 -> Product/2
  radius/1 -> Product1/1
  PS-Simulink Converter/1 -> Transfer Fcn/1
  Transfer Fcn/1 -> Product1/2
  connections:
  Simulink-PS Converter/RConn1 -- Side Force/RConn1
  PS-Simulink Converter/LConn1 -- Angular Acceleration/RConn1

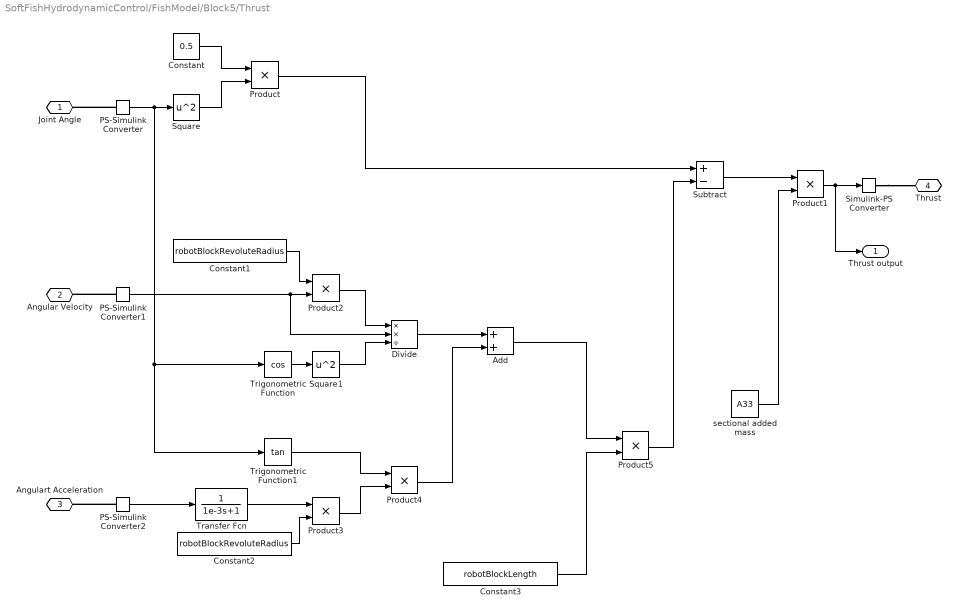
== system SoftFishHydrodynamicControl/FishModel/Block5/Thrust ==
  Add : Sum
  Constant : Constant  Value=0.5
  Constant1 : Constant  Value=robotBlockRevoluteRadius
  Constant2 : Constant  Value=robotBlockRevoluteRadius
  Constant3 : Constant  Value=robotBlockLength
  Divide : Product  Inputs=**/
  PS-Simulink Converter : nesl_utility/PS-Simulink Converter  PhysicalDomain=network_engine_domain  SubClassName=ps_output  LeftPortType=input  RightPortType=output  PseudoPeriodic=off  Frequencies=[]  Unit=inherit  AffineConversion=off
  PS-Simulink Converter1 : nesl_utility/PS-Simulink Converter  PhysicalDomain=network_engine_domain  SubClassName=ps_output  LeftPortType=input  RightPortType=output  PseudoPeriodic=off  Frequencies=[]  Unit=inherit  AffineConversion=off
  PS-Simulink Converter2 : nesl_utility/PS-Simulink Converter  PhysicalDomain=network_engine_domain  SubClassName=ps_output  LeftPortType=input  RightPortType=output  PseudoPeriodic=off  Frequencies=[]  Unit=inherit  AffineConversion=off
  Product{,1..5} (6 alike) : Product
  Simulink-PS Converter : nesl_utility/Simulink-PS Converter  PhysicalDomain=network_engine_domain  SubClassName=ps_input  LeftPortType=input  RightPortType=output  PseudoPeriodic=off  Frequencies=[]  NoiseDistribution=none  NoiseParameters=[]  Unit=1  AffineConversion=off  FilteringAndDerivatives=provide  SimscapeFilterOrder=1  InputFilterTimeConstant=0.001  UdotUserProvided=0
  Square : Math  Operator=square  SaturateOnIntegerOverflow=on
  Square1 : Math  Operator=square  SaturateOnIntegerOverflow=on
  Subtract : Sum  Inputs=+-
  Transfer Fcn : TransferFcn  Denominator=[1e-3 1]
  Trigonometric Function : Trigonometry  Operator=cos
  Trigonometric Function1 : Trigonometry  Operator=tan
  sectional added mass : Constant  Value=A33
  Joint Angle : PMIOPort  Side=Left
  Angular Velocity : PMIOPort  Port=2  Side=Left
  Angulart Acceleration : PMIOPort  Port=3  Side=Left
  Thrust : PMIOPort  Port=4  Side=Right
  Thrust output : Outport
  wires:
  Constant/1 -> Product/1
  Square/1 -> Product/2
  sectional added mass/1 -> Product1/2
  Subtract/1 -> Product1/1
  Product/1 -> Subtract/1
  Trigonometric Function/1 -> Square1/1
  PS-Simulink Converter1/1 -> Divide/2, Product2/2
  Product2/1 -> Divide/1
  Square1/1 -> Divide/3
  Divide/1 -> Add/1
  Constant1/1 -> Product2/1
  PS-Simulink Converter2/1 -> Transfer Fcn/1
  Constant2/1 -> Product3/2
  Product3/1 -> Product4/2
  Trigonometric Function1/1 -> Product4/1
  Product4/1 -> Add/2
  Add/1 -> Product5/1
  Constant3/1 -> Product5/2
  Product5/1 -> Subtract/2
  Product1/1 -> Thrust output/1, Simulink-PS Converter/1
  Transfer Fcn/1 -> Product3/1
  PS-Simulink Converter/1 -> Trigonometric Function1/1, Trigonometric Function/1, Square/1
  connections:
  PS-Simulink Converter/LConn1 -- Joint Angle/RConn1
  PS-Simulink Converter2/LConn1 -- Angulart Acceleration/RConn1
  PS-Simulink Converter1/LConn1 -- Angular Velocity/RConn1
  Simulink-PS Converter/RConn1 -- Thrust/RConn1

== matlab function SoftFishHydrodynamicControl/FishModel/MATLAB Function ==
  data: inputPressureAmplitude input; inputFrequency input; inputPressureLeft output; inputTime input; inputPressureRight output
function [inputPressureLeft, inputPressureRight] = generateSquareWave(inputPressureAmplitude, inputFrequency, inputTime)
    inputPressureLeft  = 0.5 * (inputPressureAmplitude * square( (2*pi*inputFrequency)*inputTime ) + inputPressureAmplitude);
    inputPressureRight = 0.5 * inputPressureAmplitude * (1-square( (2*pi*inputFrequency)*inputTime ));
end
